simulink model "quadsim"  (Simulink 7.7)
settings: Solver=ode45  StartTime=0.0  StopTime=50  RelTol=1e-3
values from neighbouring files (symbols this model uses):
  b = 9.7575e-6    (= 9.7575e-06)    [ForcesTest.m]    (also in QuadDynamics.m = 9.937e-09; QuadDynamicsC.m = 1.7246e-06; Quadparameters.m = 3.13e-05; quadparam.m = 3.13e-05)
  d = 7.5*10^(-7)    (= 7.5e-07)    [Quadparameters.m]    (also in quadparam.m)
  g = 9.81    [ForcesTest.m]    (also in QuadDynamics.m; QuadDynamicsC.m; Quadparameters.m; quadparam.m)
  Ix = 7.5*10^(-3)    (= 0.0075)    [Quadparameters.m]    (also in quadparam.m)
  Iy = 7.5*10^(-3)    (= 0.0075)    [Quadparameters.m]    (also in quadparam.m)
  Iz = 1.3*10^(-2)    (= 0.013)    [Quadparameters.m]    (also in quadparam.m)
  Jr = 6.5*10^(-5)    (= 6.5e-05)    [Quadparameters.m]    (also in quadparam.m = 0.100065)
  kdp = 0.4    [Quadparameters.m]    (also in quadparam.m)
  kdps = 0.4    [Quadparameters.m]    (also in quadparam.m)
  kdt = 0.4    [Quadparameters.m]    (also in quadparam.m)
  kdz = 20    [Quadparameters.m]    (also in quadparam.m = 80)
  kpp = 0.8    [Quadparameters.m]    (also in quadparam.m)
  kpps = 1    [Quadparameters.m]    (also in quadparam.m)
  kpt = 1.2    [Quadparameters.m]    (also in quadparam.m)
  kpz = 100    [Quadparameters.m]    (also in quadparam.m)
  l = 0.3    [ForcesTest.m]    (also in QuadDynamics.m = 0.254; QuadDynamicsC.m = 0.254; Quadparameters.m = 0.23; quadparam.m = 0.5)
  m = 1.282    [ForcesTest.m]    (also in QuadDynamics.m = 1.284; QuadDynamicsC.m = 1.284; Quadparameters.m = 0.65; quadparam.m = 0.65)
libraries: simulink x1
settings Model: Creator=abdelrazzak.merheb  LastModifiedBy=Alexey
settings DebuggingCC: StrictBusMsg=Warning

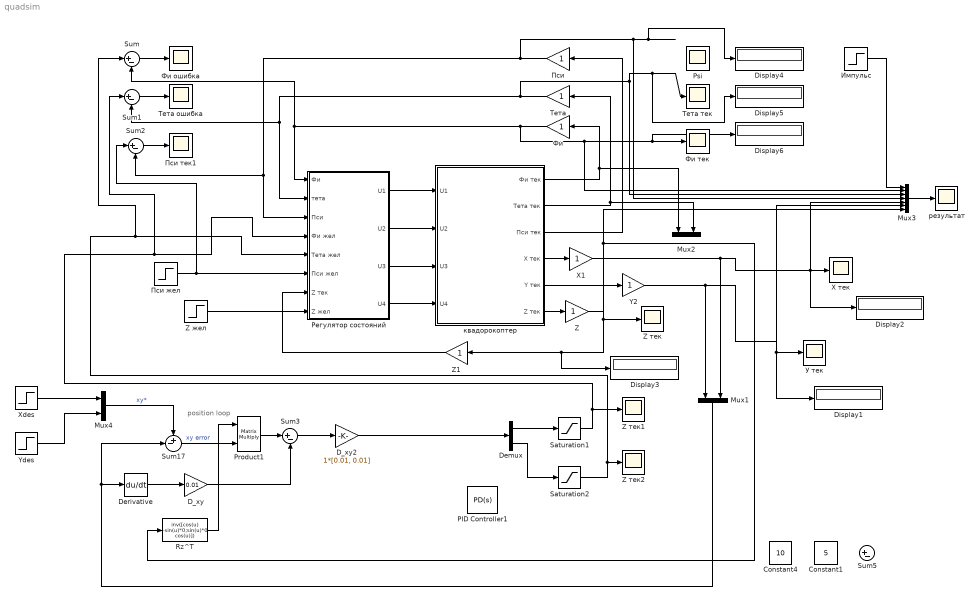
== system quadsim ==
  note: position
      | loop
  Constant1 : Constant  Value=5
  Constant4 : Constant  Value=10
  D_xy : Gain  Gain=0.01
  D_xy2 : Gain  Gain=1*[0.01, 0.01]
  Demux : Demux  Outputs=2
  Derivative : Derivative
  Display{1..6} (6 alike) : Display
  Mux1 : Mux  Inputs=2
  Mux2 : Mux  Inputs=2
  Mux3 : Mux  Inputs=7
  Mux4 : Mux  Inputs=2
  PID Controller1 : simulink/Continuous/PID Controller  SystemSampleTime=-1  Controller=PD  TimeDomain=Continuous-time  SampleTime=1  IntegratorMethod=Forward Euler  FilterMethod=Forward Euler  Form=Parallel  P=1  I=1  D=5  N=100  InitialConditionSource=internal  InitialConditionForIntegrator=0  InitialConditionForFilter=0  ExternalReset=none  LimitOutput=off  UpperSaturationLimit=inf  LowerSaturationLimit=-inf  LinearizeAsGain=off  AntiWindupMode=none  Kb=1  TrackingMode=off  Kt=1  PParamMin=[]  PParamMax=[]  IParamMin=[]  IParamMax=[]  DParamMin=[]  DParamMax=[]  NParamMin=[]  NParamMax=[]  KbParamMin=[]  KbParamMax=[]  KtParamMin=[]  KtParamMax=[]  POutMin=[]  POutMax=[]  IOutMin=[]  IOutMax=[]  DOutMin=[]  DOutMax=[]  NOutMin=[]  NOutMax=[]  KbOutMin=[]  KbOutMax=[]  KtOutMin=[]  KtOutMax=[]  IntegratorOutMin=[]  IntegratorOutMax=[]  FilterOutMin=[]  FilterOutMax=[]  SumOutMin=[]  SumOutMax=[]  SumI1OutMin=[]  SumI1OutMax=[]  SumI2OutMin=[]  SumI2OutMax=[]  SumI3OutMin=[]  SumI3OutMax=[]  SumDOutMin=[]  SumDOutMax=[]  SaturationOutMin=[]  SaturationOutMax=[]  IntegratorContinuousStateAttributes=''  IntegratorStateMustResolveToSignalObject=off  IntegratorRTWStateStorageClass=Auto  FilterContinuousStateAttributes=''  FilterStateMustResolveToSignalObject=off  FilterRTWStateStorageClass=Auto
  Product1 : Product  Multiplication=Matrix(*)  RndMeth=Zero
  Psi : Scope
      settings: YMin=-8.4  YMax=-7.6  SaveName=ScopeData2
  Rz^T : MATLABFcn  MATLABFcn=inv([cos(u) -sin(u)*0;sin(u)*0 cos(u)])  OutputDimensions=[2 2]  Output1D=off
  Saturation1 : Saturate  ZeroCross=off
  Saturation2 : Saturate  ZeroCross=off
  Sum{,1..3,5} (5 alike) : Sum  Inputs=|+-
  Sum17 : Sum  Inputs=+-|
  X тек : Scope
      settings: TimeRange=13.87832699619772  YMin=8.4  YMax=8.485  SaveName=ScopeData6
  X1 : Gain
  Xdes : Step  Time=10  After=3  SampleTime=0
  Y2 : Gain
  Ydes : Step  After=0  SampleTime=0
  Z : Gain
  Z жел : Step  After=2  SampleTime=0
  Z тек : Scope
      settings: YMin=21.8  YMax=22.05  SaveName=ScopeData4
  Z тек1 : Scope
      settings: YMin=0.50025  YMax=0.5025  SaveName=ScopeData8
  Z тек2 : Scope
      settings: YMin=1.08342  YMax=1.08355  SaveName=ScopeData12
  Z1 : Gain
  Импульс : Step  SampleTime=0
  Пси : Gain
  Пси жел : Step  After=0  SampleTime=0
  Пси тек1 : Scope
      settings: SaveName=ScopeData11
  Регулятор состояний : Subsystem
  Тета : Gain
  Тета ошибка : Scope
      settings: SaveName=ScopeData10
  Тета тек : Scope
  У тек : Scope
      settings: TimeRange=50  YMin=0  YMax=3500  SaveName=ScopeData7
  Фи : Gain
  Фи ошибка : Scope
      settings: SaveName=ScopeData9
  Фи тек : Scope
  квадорокоптер : Subsystem
  результат : Scope
      settings: SaveName=ScopeData3
  wires:
  Регулятор состояний/1(U1) -> квадорокоптер/1(U1)
  Регулятор состояний/2(U2) -> квадорокоптер/2(U2)
  Регулятор состояний/3(U3) -> квадорокоптер/3(U3)
  Регулятор состояний/4(U4) -> квадорокоптер/4(U4)
  квадорокоптер/6(Z тек) -> Z/1
  квадорокоптер/1(Фи тек) -> Фи/1, Mux2/1
  квадорокоптер/2(Тета тек) -> Тета/1, Mux2/2
  квадорокоптер/3(Пси тек) -> Пси/1
  Пси жел/1 -> Регулятор состояний/6(Пси жел), Sum2/1
  Z жел/1 -> Регулятор состояний/8(Z жел)
  квадорокоптер/4(X тек) -> X1/1
  квадорокоптер/5(Y тек) -> Y2/1
  Z/1 -> Z тек/1, Display3/1, Z1/1, Rz^T/1, Mux3/7
  Пси/1 -> Mux3/4, ?Psi тек/1, Display4/1, Регулятор состояний/3(Пси), Sum2/2
  Тета/1 -> Mux3/3, Тета тек/1, Display5/1, Регулятор состояний/2(тета), Sum1/2
  Фи/1 -> Mux3/2, Фи тек/1, Display6/1, Регулятор состояний/1(Фи), Sum/2
  Импульс/1 -> Mux3/1
  Mux3/1 -> результат/1
  Z1/1 -> Регулятор состояний/7(Z тек)
  X1/1 -> X тек/1, Display2/1, Mux3/5, Mux1/2
  Y2/1 -> У тек/1, Display1/1, Mux3/6, Mux1/1
  Sum/1 -> Фи ошибка/1
  Sum1/1 -> Тета ошибка/1
  Sum2/1 -> Пси тек1/1
  Mux4/1 -> Sum17/1  "xy*"
  Rz^T/1 -> Product1/1
  Sum17/1 -> Product1/2  "xy error"
  Mux1/1 -> Sum17/2, Derivative/1
  Demux/1 -> Saturation1/1
  Product1/1 -> Sum3/1
  D_xy/1 -> Sum3/2
  Derivative/1 -> D_xy/1
  Demux/2 -> Saturation2/1
  Xdes/1 -> Mux4/1
  Ydes/1 -> Mux4/2
  Saturation1/1 -> Sum1/1, Регулятор состояний/4(Фи жел), Z тек1/1
  Saturation2/1 -> Sum/1, Регулятор состояний/5(Тета жел), Z тек2/1
  Sum3/1 -> D_xy2/1
  D_xy2/1 -> Demux/1

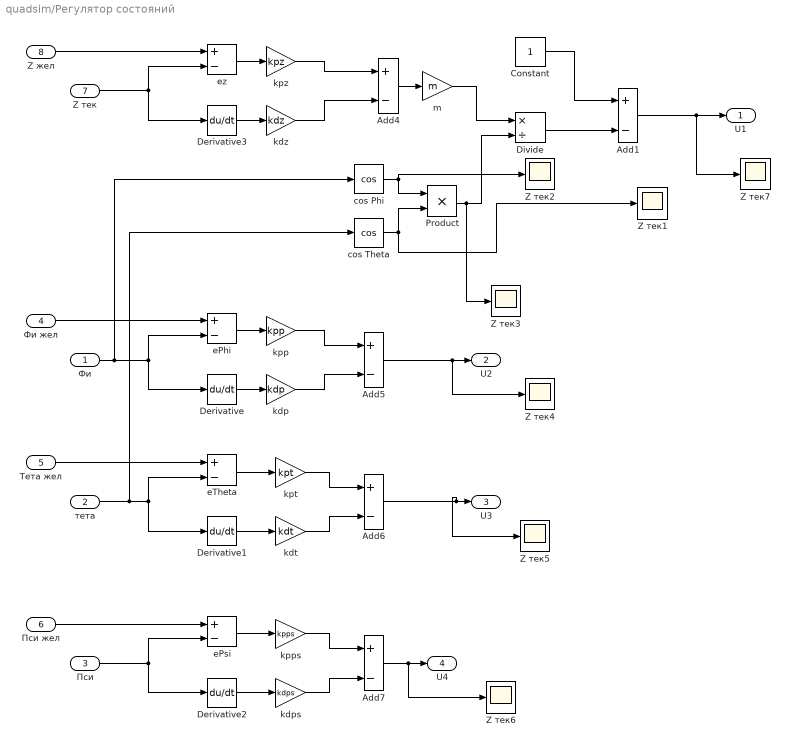
== system quadsim/Регулятор состояний ==
  Фи : Inport
  тета : Inport  Port=2
  Пси : Inport  Port=3
  Фи жел : Inport  Port=4
  Тета жел : Inport  Port=5
  Пси жел : Inport  Port=6
  Z тек : Inport  Port=7
  Z жел : Inport  Port=8
  Add{1,4..7} (5 alike) : Sum  Inputs=+-
  Constant : Constant
  Derivative{,1..3} (4 alike) : Derivative
  Divide : Product  Inputs=*/
  Product : Product  RndMeth=Zero
  Z тек{1..7} (7 alike) : Scope
      Z тек1 settings: YMin=1.08342  YMax=1.08355  SaveName=ScopeData13
      Z тек2 settings: YMin=1.08342  YMax=1.08355  SaveName=ScopeData14
      Z тек3 settings: YMin=1.08342  YMax=1.08355  SaveName=ScopeData15
      Z тек4 settings: YMin=1.08342  YMax=1.08355  SaveName=ScopeData18
      Z тек5 settings: YMin=1.08342  YMax=1.08355  SaveName=ScopeData19
      Z тек6 settings: YMin=1.08342  YMax=1.08355  SaveName=ScopeData20
      Z тек7 settings: YMin=-1000  YMax=-995  SaveName=ScopeData21
  cos Phi : Trigonometry  Operator=cos
  cos Theta : Trigonometry  Operator=cos
  ePhi : Sum  Inputs=+-
  ePsi : Sum  Inputs=+-
  eTheta : Sum  Inputs=+-
  ez : Sum  Inputs=+-
  kdp : Gain  Gain=kdp
  kdps : Gain  Gain=kdps
  kdt : Gain  Gain=kdt
  kdz : Gain  Gain=kdz
  kpp : Gain  Gain=kpp
  kpps : Gain  Gain=kpps
  kpt : Gain  Gain=kpt
  kpz : Gain  Gain=kpz
  m : Gain  Gain=m
  U1 : Outport
  U2 : Outport  Port=2
  U3 : Outport  Port=3
  U4 : Outport  Port=4
  wires:
  Фи/1 -> Derivative/1, ePhi/2, cos Phi/1
  тета/1 -> Derivative1/1, eTheta/2, cos Theta/1
  Пси/1 -> Derivative2/1, ePsi/2
  Фи жел/1 -> ePhi/1
  Тета жел/1 -> eTheta/1
  Пси жел/1 -> ePsi/1
  ePhi/1 -> kpp/1
  Derivative/1 -> kdp/1
  eTheta/1 -> kpt/1
  Derivative1/1 -> kdt/1
  ePsi/1 -> kpps/1
  Derivative2/1 -> kdps/1
  Z тек/1 -> Derivative3/1, ez/2
  Z жел/1 -> ez/1
  ez/1 -> kpz/1
  Derivative3/1 -> kdz/1
  kpz/1 -> Add4/1
  kdz/1 -> Add4/2
  kpp/1 -> Add5/1
  kdp/1 -> Add5/2
  Add5/1 -> U2/1, Z тек4/1
  kpt/1 -> Add6/1
  kdt/1 -> Add6/2
  Add6/1 -> U3/1, Z тек5/1
  kpps/1 -> Add7/1
  kdps/1 -> Add7/2
  Add7/1 -> U4/1, Z тек6/1
  cos Phi/1 -> Product/1, Z тек2/1
  cos Theta/1 -> Product/2, Z тек1/1
  Add4/1 -> m/1
  Product/1 -> Divide/2, Z тек3/1
  Divide/1 -> Add1/2
  m/1 -> Divide/1
  Constant/1 -> Add1/1
  Add1/1 -> U1/1, Z тек7/1

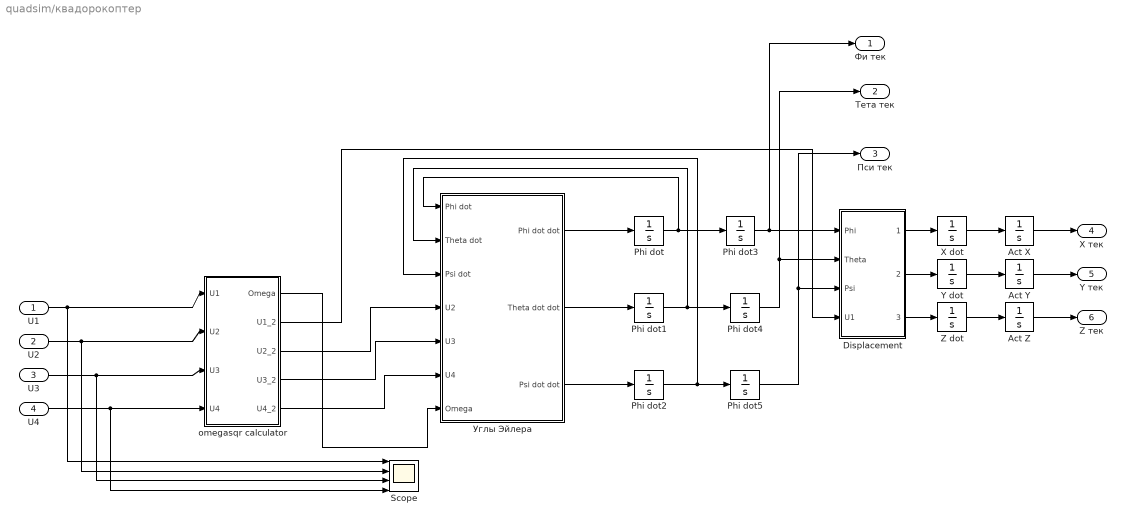
== system quadsim/квадорокоптер ==
  U1 : Inport
  U2 : Inport  Port=2
  U3 : Inport  Port=3
  U4 : Inport  Port=4
  Act X : Integrator
  Act Y : Integrator
  Act Z : Integrator
  Displacement : Subsystem
  Phi dot : Integrator
  Phi dot{1..5} (5 alike) : Integrator  ZeroCross=off
  Scope : Scope  NumInputPorts=4
      settings: YMin=6.35~-0.15~-0.075~-5  YMax=6.85~0.15~0.075~5  SaveName=ScopeData5
  X dot : Integrator
  Y dot : Integrator
  Z dot : Integrator
  omegasqr calculator : Subsystem
  Углы Эйлера : Subsystem
  Фи тек : Outport
  Тета тек : Outport  Port=2
  Пси тек : Outport  Port=3
  X тек : Outport  Port=4
  Y тек : Outport  Port=5
  Z тек : Outport  Port=6
  wires:
  Углы Эйлера/1(Phi dot dot) -> Phi dot/1
  Углы Эйлера/2(Theta dot dot) -> Phi dot1/1
  Углы Эйлера/3(Psi dot dot) -> Phi dot2/1
  Phi dot/1 -> Углы Эйлера/1(Phi dot), Phi dot3/1
  Phi dot1/1 -> Углы Эйлера/2(Theta dot), Phi dot4/1
  Phi dot2/1 -> Углы Эйлера/3(Psi dot), Phi dot5/1
  omegasqr calculator/3(U2_2) -> Углы Эйлера/4(U2)
  omegasqr calculator/4(U3_2) -> Углы Эйлера/5(U3)
  omegasqr calculator/5(U4_2) -> Углы Эйлера/6(U4)
  omegasqr calculator/1(Omega) -> Углы Эйлера/7(Omega)
  Phi dot3/1 -> Displacement/1(Phi), Фи тек/1
  Phi dot4/1 -> Displacement/2(Theta), Тета тек/1
  Phi dot5/1 -> Displacement/3(Psi), Пси тек/1
  omegasqr calculator/2(U1_2) -> Displacement/4(U1)
  Displacement/1(x dotdot) -> X dot/1
  X dot/1 -> Act X/1
  Y dot/1 -> Act Y/1
  Displacement/2(y dotdot) -> Y dot/1
  Z dot/1 -> Act Z/1
  Displacement/3(z dotdot) -> Z dot/1
  Act X/1 -> X тек/1
  Act Y/1 -> Y тек/1
  Act Z/1 -> Z тек/1
  U1/1 -> omegasqr calculator/1(U1), Scope/1
  U2/1 -> omegasqr calculator/2(U2), Scope/2
  U3/1 -> omegasqr calculator/3(U3), Scope/3
  U4/1 -> omegasqr calculator/4(U4), Scope/4

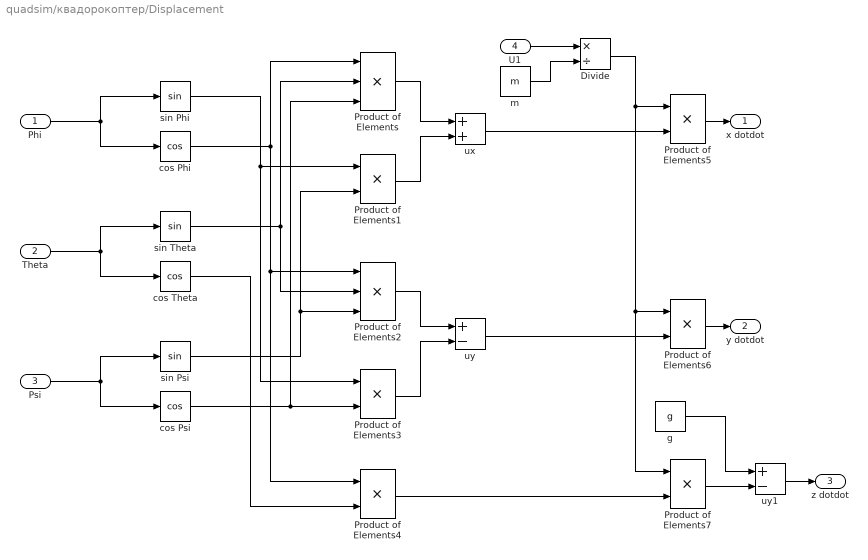
== system quadsim/квадорокоптер/Displacement ==
  Phi : Inport
  Theta : Inport  Port=2
  Psi : Inport  Port=3
  U1 : Inport  Port=4
  Divide : Product  Inputs=*/
  Product of Elements : Product  Inputs=3
  Product of Elements{1,3..7} (6 alike) : Product
  Product of Elements2 : Product  Inputs=3
  cos Phi : Trigonometry  Operator=cos
  cos Psi : Trigonometry  Operator=cos
  cos Theta : Trigonometry  Operator=cos
  g : Constant  Value=g
  m : Constant  Value=m
  sin Phi : Trigonometry
  sin Psi : Trigonometry
  sin Theta : Trigonometry
  ux : Sum
  uy : Sum  Inputs=+-
  uy1 : Sum  Inputs=+-
  x dotdot : Outport
  y dotdot : Outport  Port=2
  z dotdot : Outport  Port=3
  wires:
  Phi/1 -> sin Phi/1, cos Phi/1
  Theta/1 -> sin Theta/1, cos Theta/1
  Psi/1 -> sin Psi/1, cos Psi/1
  sin Theta/1 -> Product of Elements/2, Product of Elements2/2
  cos Psi/1 -> Product of Elements/3, Product of Elements3/2
  cos Phi/1 -> Product of Elements/1, Product of Elements2/1, Product of Elements4/1
  sin Phi/1 -> Product of Elements1/1, Product of Elements3/1
  sin Psi/1 -> Product of Elements1/2, Product of Elements2/3
  Product of Elements/1 -> ux/1
  Product of Elements1/1 -> ux/2
  ux/1 -> Product of Elements5/2
  Product of Elements2/1 -> uy/1
  Product of Elements3/1 -> uy/2
  uy/1 -> Product of Elements6/2
  cos Theta/1 -> Product of Elements4/2
  Product of Elements4/1 -> Product of Elements7/2
  U1/1 -> Divide/1
  m/1 -> Divide/2
  Divide/1 -> Product of Elements5/1, Product of Elements6/1, Product of Elements7/1
  Product of Elements5/1 -> x dotdot/1
  Product of Elements6/1 -> y dotdot/1
  uy1/1 -> z dotdot/1
  Product of Elements7/1 -> uy1/2
  g/1 -> uy1/1

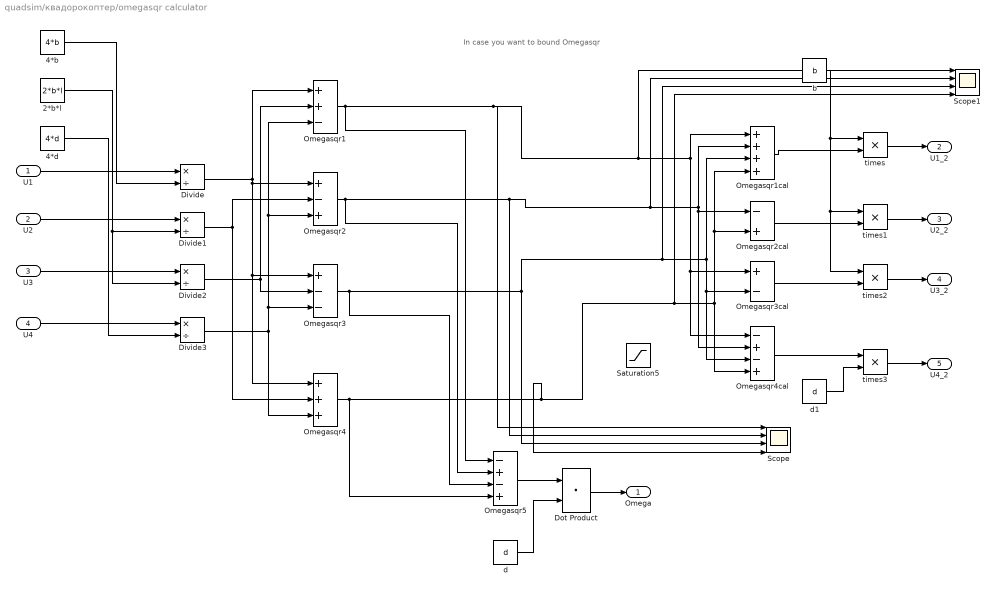
== system quadsim/квадорокоптер/omegasqr calculator ==
  note: In case you want to bound Omegasqr
  U1 : Inport
  U2 : Inport  Port=2
  U3 : Inport  Port=3
  U4 : Inport  Port=4
  2*b*l : Constant  Value=2*b*l
  4*b : Constant  Value=4*b
  4*d : Constant  Value=4*d
  Divide{,1..3} (4 alike) : Product  Inputs=*/
  Dot Product : DotProduct  InputSameDT=on  OutDataTypeStr=Inherit: Inherit via internal rule
  Omegasqr1 : Sum  Inputs=++-
  Omegasqr1cal : Sum  Inputs=++++
  Omegasqr2 : Sum  Inputs=+-+
  Omegasqr2cal : Sum  Inputs=-+
  Omegasqr3 : Sum  Inputs=+--
  Omegasqr3cal : Sum  Inputs=+-
  Omegasqr4 : Sum  Inputs=+++
  Omegasqr4cal : Sum  Inputs=-+-+
  Omegasqr5 : Sum  Inputs=-+-+
  Saturation5 : Saturate  UpperLimit=1000000  LowerLimit=0  ZeroCross=off
  Scope : Scope  NumInputPorts=4
      settings: YMin=6.35~-0.15~-0.075~-5  YMax=6.85~0.15~0.075~5  SaveName=ScopeData16
  Scope1 : Scope  NumInputPorts=4
      settings: YMin=6.35~-0.15~-0.075~-5  YMax=6.85~0.15~0.075~5  SaveName=ScopeData17
  b : Constant  Value=b
  d : Constant  Value=d
  d1 : Constant  Value=d
  times{,1..3} (4 alike) : Product  Inputs=**
  Omega : Outport
  U1_2 : Outport  Port=2
  U2_2 : Outport  Port=3
  U3_2 : Outport  Port=4
  U4_2 : Outport  Port=5
  wires:
  U1/1 -> Divide/1
  4*b/1 -> Divide/2
  U2/1 -> Divide1/1
  2*b*l/1 -> Divide1/2, Divide2/2
  U3/1 -> Divide2/1
  U4/1 -> Divide3/1
  4*d/1 -> Divide3/2
  Divide/1 -> Omegasqr1/1, Omegasqr2/1, Omegasqr3/1, Omegasqr4/1
  Divide2/1 -> Omegasqr1/2, Omegasqr3/2
  Divide3/1 -> Omegasqr1/3, Omegasqr2/3, Omegasqr3/3, Omegasqr4/3
  Divide1/1 -> Omegasqr2/2, Omegasqr4/2
  Omegasqr1/1 -> Omegasqr5/1, Scope/1, Omegasqr1cal/1, Omegasqr3cal/1, Omegasqr4cal/1, Scope1/1
  Omegasqr2/1 -> Omegasqr5/2, Scope/2, Omegasqr1cal/2, Omegasqr2cal/1, Omegasqr4cal/2, Scope1/2
  Omegasqr3/1 -> Omegasqr5/3, Scope/3, Omegasqr1cal/3, Omegasqr3cal/2, Omegasqr4cal/3, Scope1/3
  Omegasqr4/1 -> Omegasqr5/4, Scope/4, Omegasqr1cal/4, Omegasqr2cal/2, Omegasqr4cal/4, Scope1/4
  Omegasqr5/1 -> Dot Product/1
  Dot Product/1 -> Omega/1
  d/1 -> Dot Product/2
  b/1 -> times/1, times1/1, times2/1
  Omegasqr1cal/1 -> times/2
  Omegasqr2cal/1 -> times1/2
  Omegasqr3cal/1 -> times2/2
  Omegasqr4cal/1 -> times3/1
  d1/1 -> times3/2
  times/1 -> U1_2/1
  times1/1 -> U2_2/1
  times3/1 -> U4_2/1
  times2/1 -> U3_2/1

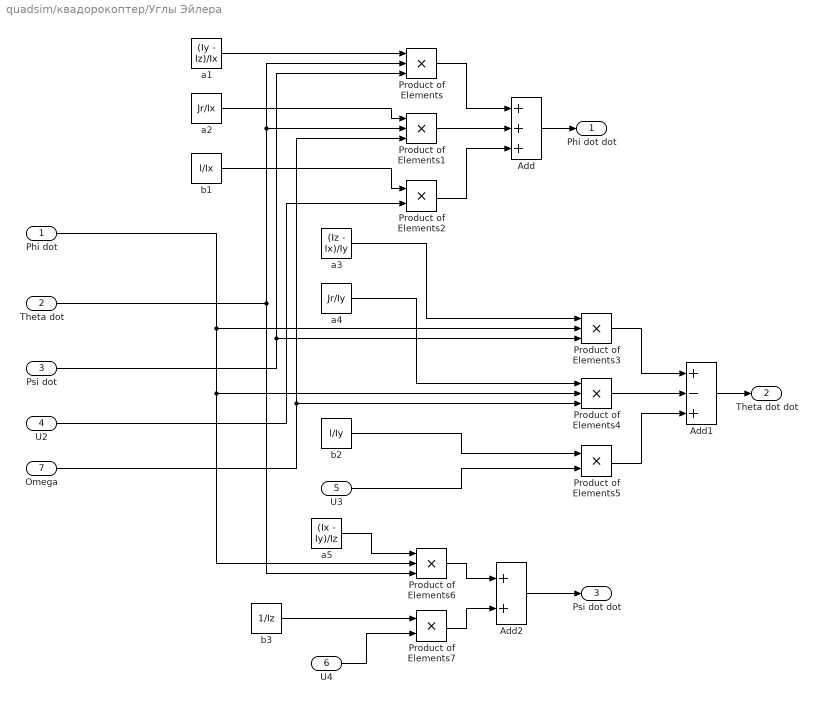
== system quadsim/квадорокоптер/Углы Эйлера ==
  Phi dot : Inport
  Theta dot : Inport  Port=2
  Psi dot : Inport  Port=3
  U2 : Inport  Port=4
  U3 : Inport  Port=5
  U4 : Inport  Port=6
  Omega : Inport  Port=7
  Add : Sum  Inputs=+++
  Add1 : Sum  Inputs=+-+
  Add2 : Sum
  Product of Elements{,1,3..4,6} (5 alike) : Product  Inputs=3
  Product of Elements2 : Product
  Product of Elements5 : Product
  Product of Elements7 : Product
  a1 : Constant  Value=(Iy - Iz)/Ix
  a2 : Constant  Value=Jr/Ix
  a3 : Constant  Value=(Iz - Ix)/Iy
  a4 : Constant  Value=Jr/Iy
  a5 : Constant  Value=(Ix - Iy)/Iz
  b1 : Constant  Value=l/Ix
  b2 : Constant  Value=l/Iy
  b3 : Constant  Value=1/Iz
  Phi dot dot : Outport
  Theta dot dot : Outport  Port=2
  Psi dot dot : Outport  Port=3
  wires:
  Product of Elements/1 -> Add/1
  Product of Elements1/1 -> Add/2
  Product of Elements2/1 -> Add/3
  Add/1 -> Phi dot dot/1
  a1/1 -> Product of Elements/1
  Theta dot/1 -> Product of Elements/2, Product of Elements1/2, Product of Elements6/3
  Psi dot/1 -> Product of Elements/3, Product of Elements3/3
  a2/1 -> Product of Elements1/1
  b1/1 -> Product of Elements2/1
  U2/1 -> Product of Elements2/2
  Omega/1 -> Product of Elements1/3, Product of Elements4/3
  Product of Elements3/1 -> Add1/1
  Product of Elements4/1 -> Add1/2
  Product of Elements5/1 -> Add1/3
  Add1/1 -> Theta dot dot/1
  a3/1 -> Product of Elements3/1
  a4/1 -> Product of Elements4/1
  b2/1 -> Product of Elements5/1
  U3/1 -> Product of Elements5/2
  Phi dot/1 -> Product of Elements3/2, Product of Elements4/2, Product of Elements6/2
  Product of Elements6/1 -> Add2/1
  Product of Elements7/1 -> Add2/2
  Add2/1 -> Psi dot dot/1
  U4/1 -> Product of Elements7/2
  b3/1 -> Product of Elements7/1
  a5/1 -> Product of Elements6/1
